simulink model "att2e"  (Simulink 6.3)
settings: Solver=FixedStepDiscrete  StartTime=0.0  StopTime=0  FixedStep=1  RelTol=1e-3
undefined symbols (not defined in the file or in its folder): att2e_att_type, att2e_dc_L2W
libraries: simulink x1, utility_lib x1
settings Model: LastModifiedBy=E700252  StrictBusMsg=None
settings DataIOCC: SaveOutput=off  SaveTime=off  SignalLoggingName=sigsOut
settings OptimizationCC: InlineInvariantSignals=on
settings DebuggingCC: SolverPrmCheckMsg=none
settings HardwareCC: TargetUnknown=on

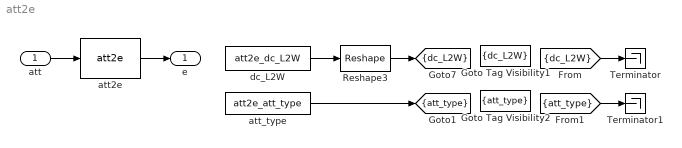
== system att2e ==
  att : Inport
  Goto Tag Visibility1 : GotoTagVisibility  GotoTag=dc_L2W
  Goto Tag Visibility2 : GotoTagVisibility  GotoTag=att_type
  Reshape3 : simulink/Math Operations/Reshape  OutputDimensionality=1-D array  OutputDimensions=[3 3]
  Terminator : Terminator
  Terminator1 : Terminator
  att2e : utility_lib/att2e  quat_IC=att2e_quat_IC
  att_type : Constant  Value=att2e_att_type
  dc_L2W : Constant  Value=att2e_dc_L2W
  e : Outport
  tag scope: att_type=scoped, dc_L2W=scoped
  wires:
  att/1 -> att2e/1
  att2e/1 -> e/1
  dc_L2W/1 -> Reshape3/1
  Reshape3/1 -> [dc_L2W]
  [dc_L2W] -> Terminator/1
  [att_type] -> Terminator1/1
  att_type/1 -> [att_type]
